simulink model "Flight_Controller_ForStudent"  (R2017b)
settings: Solver=FixedStepDiscrete  StartTime=0.0  StopTime=10.0  FixedStep=Ts  RelTol=1e-3
undefined symbols (not defined in the file or in its folder): Actuators, Gear, Lim, Sim_trimInput, TP_Euler, Ts
libraries: simulink x4
settings Model: Creator=zht  LastModifiedBy=One

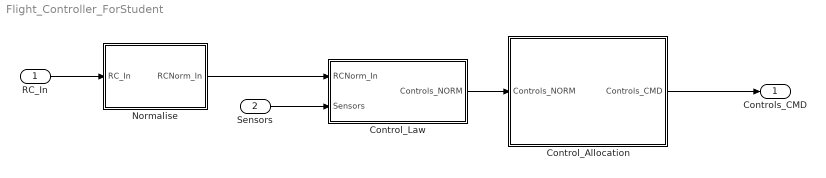
== system Flight_Controller_ForStudent ==
  RC_In : Inport  OutDataTypeStr=Bus: RC_In_BUS
  Sensors : Inport  Port=2  OutDataTypeStr=Bus: Sensors_BUS
  Control_Allocation : Subsystem
  Control_Law : Subsystem
  Normalise : Subsystem
  Controls_CMD : Outport  OutDataTypeStr=Bus: Controls_CMD_BUS
  wires:
  Control_Allocation/1(Controls_CMD) -> Controls_CMD/1
  Control_Law/1(Controls_NORM) -> Control_Allocation/1(Controls_NORM)
  Sensors/1 -> Control_Law/2(Sensors)
  RC_In/1 -> Normalise/1(RC_In)
  Normalise/1(RCNorm_In) -> Control_Law/1(RCNorm_In)

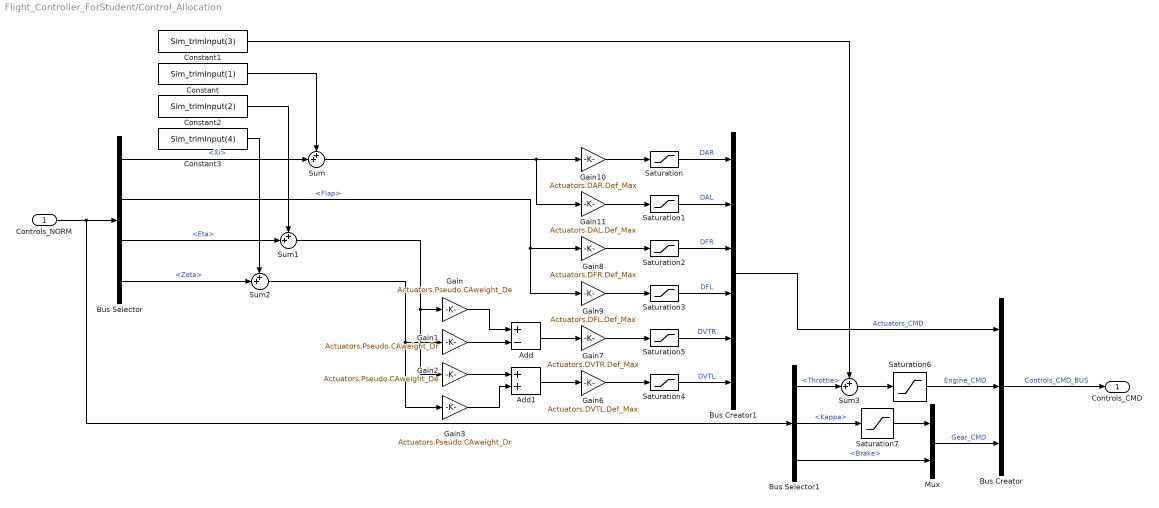
== system Flight_Controller_ForStudent/Control_Allocation ==
  Controls_NORM : Inport
  Add : Sum  Inputs=+-
  Add1 : Sum
  Bus Creator : BusCreator  Inputs=3  OutDataTypeStr=Bus: Controls_CMD_BUS
  Bus Creator1 : BusCreator  Inputs=6  OutDataTypeStr=Bus: Actuators_CMD_BUS
  Bus Selector : BusSelector  OutputSignals=Xi,Flap,Eta,Zeta
  Bus Selector1 : BusSelector  OutputSignals=Throttle,Kappa,Brake
  Constant : Constant  Value=Sim_trimInput(1)
  Constant1 : Constant  Value=Sim_trimInput(3)
  Constant2 : Constant  Value=Sim_trimInput(2)
  Constant3 : Constant  Value=Sim_trimInput(4)
  Gain : Gain  Gain=Actuators.Pseudo.CAweight_De
  Gain1 : Gain  Gain=Actuators.Pseudo.CAweight_Dr
  Gain10 : Gain  Gain=Actuators.DAR.Def_Max
  Gain11 : Gain  Gain=Actuators.DAL.Def_Max
  Gain2 : Gain  Gain=Actuators.Pseudo.CAweight_De
  Gain3 : Gain  Gain=Actuators.Pseudo.CAweight_Dr
  Gain6 : Gain  Gain=Actuators.DVTL.Def_Max
  Gain7 : Gain  Gain=Actuators.DVTR.Def_Max
  Gain8 : Gain  Gain=Actuators.DFR.Def_Max
  Gain9 : Gain  Gain=Actuators.DFL.Def_Max
  Mux : Mux  Inputs=2
  Saturation : Saturate  UpperLimit=Actuators.DAR.Def_Max  LowerLimit=Actuators.DAR.Def_Min
  Saturation1 : Saturate  UpperLimit=Actuators.DAL.Def_Max  LowerLimit=Actuators.DAL.Def_Min
  Saturation2 : Saturate  UpperLimit=Actuators.DFR.Def_Max  LowerLimit=Actuators.DFR.Def_Min
  Saturation3 : Saturate  UpperLimit=Actuators.DAL.Def_Max  LowerLimit=Actuators.DAL.Def_Min
  Saturation4 : Saturate  UpperLimit=Actuators.DVTL.Def_Max  LowerLimit=Actuators.DVTL.Def_Min
  Saturation5 : Saturate  UpperLimit=Actuators.DVTR.Def_Max  LowerLimit=Actuators.DVTR.Def_Min
  Saturation6 : Saturate  UpperLimit=1  LowerLimit=0
  Saturation7 : Saturate  UpperLimit=Gear.NoseStrut.Def_Max  LowerLimit=-Gear.NoseStrut.Def_Max
  Sum{,1..3} (4 alike) : Sum  Inputs=++|
  Controls_CMD : Outport  OutDataTypeStr=Bus: Controls_CMD_BUS
  wires:
  Bus Creator/1 -> Controls_CMD/1  "Controls_CMD_BUS"
  Bus Creator1/1 -> Bus Creator/1  "Actuators_CMD"
  Mux/1 -> Bus Creator/3  "Gear_CMD"
  Controls_NORM/1 -> Bus Selector1/1, Bus Selector/1
  Gain2/1 -> Add1/1
  Gain3/1 -> Add1/2
  Gain1/1 -> Add/2
  Gain/1 -> Add/1
  Saturation/1 -> Bus Creator1/1  "DAR"
  Saturation1/1 -> Bus Creator1/2  "DAL"
  Add/1 -> Gain7/1
  Bus Selector/2 -> Gain8/1, Gain9/1  "<Flap>"
  Saturation2/1 -> Bus Creator1/3  "DFR"
  Saturation3/1 -> Bus Creator1/4  "DFL"
  Add1/1 -> Gain6/1
  Saturation5/1 -> Bus Creator1/5  "DVTR"
  Saturation4/1 -> Bus Creator1/6  "DVTL"
  Saturation6/1 -> Bus Creator/2  "Engine_CMD"
  Bus Selector1/2 -> Saturation7/1  "<Kappa>"
  Bus Selector1/3 -> Mux/2  "<Brake>"
  Saturation7/1 -> Mux/1
  Gain6/1 -> Saturation4/1
  Gain7/1 -> Saturation5/1
  Gain8/1 -> Saturation2/1
  Gain9/1 -> Saturation3/1
  Gain10/1 -> Saturation/1
  Gain11/1 -> Saturation1/1
  Sum/1 -> Gain10/1, Gain11/1
  Sum1/1 -> Gain2/1, Gain/1
  Sum2/1 -> Gain3/1, Gain1/1
  Sum3/1 -> Saturation6/1
  Constant1/1 -> Sum3/1
  Constant2/1 -> Sum1/1
  Constant/1 -> Sum/1
  Constant3/1 -> Sum2/1
  Bus Selector/1 -> Sum/2  "<Xi>"
  Bus Selector/3 -> Sum1/2  "<Eta>"
  Bus Selector/4 -> Sum2/2  "<Zeta>"
  Bus Selector1/1 -> Sum3/2  "<Throttle>"

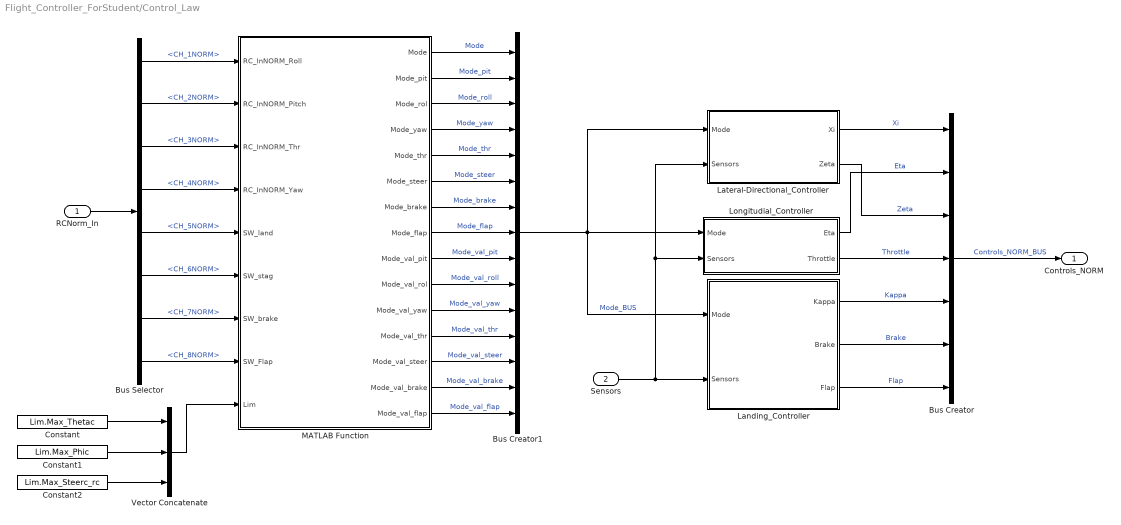
== system Flight_Controller_ForStudent/Control_Law ==
  RCNorm_In : Inport  OutDataTypeStr=Bus: RCNorm_In_BUS
  Sensors : Inport  Port=2  OutDataTypeStr=Bus: Sensors_BUS
  Bus Creator : BusCreator  Inputs=7
  Bus Creator1 : BusCreator  Inputs=15  OutDataTypeStr=Bus: Mode_BUS  NonVirtualBus=on
  Bus Selector : BusSelector  OutputSignals=CH_1NORM,CH_2NORM,CH_3NORM,CH_4NORM,CH_5NORM,CH_6NORM,CH_7NORM,CH_8NORM
  Constant : Constant  Value=Lim.Max_Thetac
  Constant1 : Constant  Value=Lim.Max_Phic
  Constant2 : Constant  Value=Lim.Max_Steerc_rc
  Landing_Controller : Subsystem
  Lateral-Directional_Controller : Subsystem
  Longitudial_Controller : Subsystem
  MATLAB Function : MATLAB Function  TreatAsAtomicUnit=on  SystemSampleTime=Ts
  Vector Concatenate : Concatenate  NumInputs=3
  Controls_NORM : Outport  OutDataTypeStr=Bus: Controls_NORM_BUS
  wires:
  Bus Creator/1 -> Controls_NORM/1  "Controls_NORM_BUS"
  Longitudial_Controller/1(Eta) -> Bus Creator/2  "Eta"
  Lateral-Directional_Controller/2(Zeta) -> Bus Creator/3  "Zeta"
  Lateral-Directional_Controller/1(Xi) -> Bus Creator/1  "Xi"
  Longitudial_Controller/2(Throttle) -> Bus Creator/4  "Throttle"
  Landing_Controller/1(Kappa) -> Bus Creator/5  "Kappa"
  Landing_Controller/2(Brake) -> Bus Creator/6  "Brake"
  Sensors/1 -> Lateral-Directional_Controller/2(Sensors), Longitudial_Controller/2(Sensors), Landing_Controller/2(Sensors)
  RCNorm_In/1 -> Bus Selector/1
  Landing_Controller/3(Flap) -> Bus Creator/7  "Flap"
  Bus Selector/1 -> MATLAB Function/1(RC_InNORM_Roll)  "<CH_1NORM>"
  Bus Selector/2 -> MATLAB Function/2(RC_InNORM_Pitch)  "<CH_2NORM>"
  Bus Selector/3 -> MATLAB Function/3(RC_InNORM_Thr)  "<CH_3NORM>"
  Bus Selector/4 -> MATLAB Function/4(RC_InNORM_Yaw)  "<CH_4NORM>"
  Bus Selector/5 -> MATLAB Function/5(SW_land)  "<CH_5NORM>"
  Bus Selector/6 -> MATLAB Function/6(SW_stag)  "<CH_6NORM>"
  Bus Selector/7 -> MATLAB Function/7(SW_brake)  "<CH_7NORM>"
  Bus Selector/8 -> MATLAB Function/8(SW_Flap)  "<CH_8NORM>"
  MATLAB Function/2(Mode_pit) -> Bus Creator1/2  "Mode_pit"
  MATLAB Function/3(Mode_rol) -> Bus Creator1/3  "Mode_roll"
  MATLAB Function/4(Mode_yaw) -> Bus Creator1/4  "Mode_yaw"
  MATLAB Function/5(Mode_thr) -> Bus Creator1/5  "Mode_thr"
  MATLAB Function/6(Mode_steer) -> Bus Creator1/6  "Mode_steer"
  MATLAB Function/7(Mode_brake) -> Bus Creator1/7  "Mode_brake"
  MATLAB Function/8(Mode_flap) -> Bus Creator1/8  "Mode_flap"
  MATLAB Function/9(Mode_val_pit) -> Bus Creator1/9  "Mode_val_pit"
  MATLAB Function/10(Mode_val_rol) -> Bus Creator1/10  "Mode_val_roll"
  MATLAB Function/11(Mode_val_yaw) -> Bus Creator1/11  "Mode_val_yaw"
  MATLAB Function/12(Mode_val_thr) -> Bus Creator1/12  "Mode_val_thr"
  MATLAB Function/13(Mode_val_steer) -> Bus Creator1/13  "Mode_val_steer"
  MATLAB Function/14(Mode_val_brake) -> Bus Creator1/14  "Mode_val_brake"
  MATLAB Function/15(Mode_val_flap) -> Bus Creator1/15  "Mode_val_flap"
  Bus Creator1/1 -> Lateral-Directional_Controller/1(Mode), Landing_Controller/1(Mode), Longitudial_Controller/1(Mode)  "Mode_BUS"
  MATLAB Function/1(Mode) -> Bus Creator1/1  "Mode"
  Constant/1 -> Vector Concatenate/1
  Constant1/1 -> Vector Concatenate/2
  Constant2/1 -> Vector Concatenate/3
  Vector Concatenate/1 -> MATLAB Function/9(Lim)

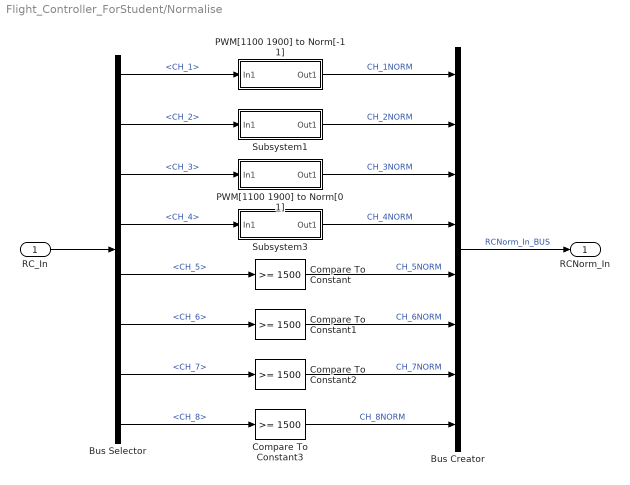
== system Flight_Controller_ForStudent/Normalise ==
  RC_In : Inport  OutDataTypeStr=Bus: RC_In_BUS
  Bus Creator : BusCreator  Inputs=8  OutDataTypeStr=Bus: RCNorm_In_BUS
  Bus Selector : BusSelector  OutputSignals=CH_1,CH_2,CH_3,CH_4,CH_5,CH_6,CH_7,CH_8
  Compare To Constant{,1..3} (4 alike) : simulink/Logic and Bit Operations/Compare To Constant  relop=>=  const=1500  OutDataTypeStr=boolean
  PWM[1100 1900] to Norm[-1 1] : Subsystem
  PWM[1100 1900] to Norm[0 1] : Subsystem
  Subsystem1 : Subsystem
  Subsystem3 : Subsystem
  RCNorm_In : Outport  OutDataTypeStr=Bus: RCNorm_In_BUS
  wires:
  RC_In/1 -> Bus Selector/1
  Bus Selector/1 -> PWM[1100 1900] to Norm[-1 1]/1(In1)  "<CH_1>"
  Bus Selector/2 -> Subsystem1/1(In1)  "<CH_2>"
  Bus Selector/3 -> PWM[1100 1900] to Norm[0 1]/1(In1)  "<CH_3>"
  Bus Selector/4 -> Subsystem3/1(In1)  "<CH_4>"
  Bus Selector/5 -> Compare To Constant/1  "<CH_5>"
  Bus Selector/6 -> Compare To Constant1/1  "<CH_6>"
  Bus Selector/7 -> Compare To Constant2/1  "<CH_7>"
  Bus Selector/8 -> Compare To Constant3/1  "<CH_8>"
  PWM[1100 1900] to Norm[-1 1]/1(Out1) -> Bus Creator/1  "CH_1NORM"
  Subsystem1/1(Out1) -> Bus Creator/2  "CH_2NORM"
  PWM[1100 1900] to Norm[0 1]/1(Out1) -> Bus Creator/3  "CH_3NORM"
  Subsystem3/1(Out1) -> Bus Creator/4  "CH_4NORM"
  Compare To Constant/1 -> Bus Creator/5  "CH_5NORM"
  Compare To Constant1/1 -> Bus Creator/6  "CH_6NORM"
  Compare To Constant2/1 -> Bus Creator/7  "CH_7NORM"
  Compare To Constant3/1 -> Bus Creator/8  "CH_8NORM"
  Bus Creator/1 -> RCNorm_In/1  "RCNorm_In_BUS"

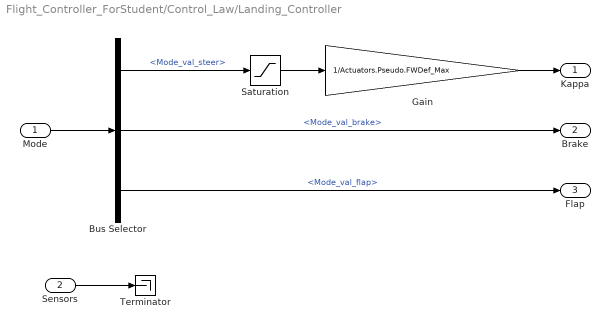
== system Flight_Controller_ForStudent/Control_Law/Landing_Controller ==
  Mode : Inport  OutDataTypeStr=Bus: Mode_BUS
  Sensors : Inport  Port=2  OutDataTypeStr=Bus: Sensors_BUS
  Bus Selector : BusSelector  OutputSignals=Mode_val_steer,Mode_val_brake,Mode_val_flap
  Gain : Gain  Gain=1/Actuators.Pseudo.FWDef_Max
  Saturation : Saturate  UpperLimit=Actuators.Pseudo.FWDef_Max  LowerLimit=-Actuators.Pseudo.FWDef_Max
  Terminator : Terminator
  Kappa : Outport
  Brake : Outport  Port=2
  Flap : Outport  Port=3
  wires:
  Mode/1 -> Bus Selector/1
  Bus Selector/1 -> Saturation/1  "<Mode_val_steer>"
  Bus Selector/2 -> Brake/1  "<Mode_val_brake>"
  Bus Selector/3 -> Flap/1  "<Mode_val_flap>"
  Sensors/1 -> Terminator/1
  Saturation/1 -> Gain/1
  Gain/1 -> Kappa/1

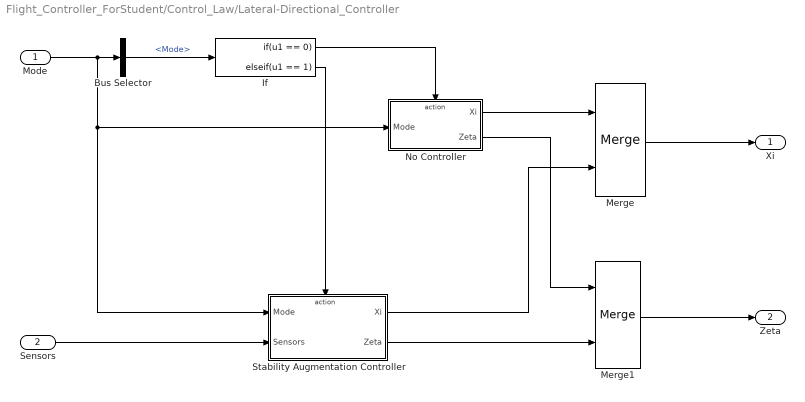
== system Flight_Controller_ForStudent/Control_Law/Lateral-Directional_Controller ==
  Mode : Inport  OutDataTypeStr=Bus: Mode_BUS
  Sensors : Inport  Port=2
  Bus Selector : BusSelector  OutputSignals=Mode
  If : If  IfExpression=u1 == 0  ElseIfExpressions=u1 == 1  ShowElse=off
  Merge : Merge
  Merge1 : Merge
  No Controller : Subsystem  TreatAsAtomicUnit=on
  Stability Augmentation Controller : Subsystem  TreatAsAtomicUnit=on
  Xi : Outport
  Zeta : Outport  Port=2
  wires:
  Sensors/1 -> Stability Augmentation Controller/2(Sensors)
  Mode/1 -> Stability Augmentation Controller/1(Mode), No Controller/1(Mode), Bus Selector/1
  Bus Selector/1 -> If/1  "<Mode>"
  If/1 -> No Controller/Action
  If/2 -> Stability Augmentation Controller/Action
  No Controller/1(Xi) -> Merge/1
  Stability Augmentation Controller/1(Xi) -> Merge/2
  No Controller/2(Zeta) -> Merge1/1
  Stability Augmentation Controller/2(Zeta) -> Merge1/2
  Merge1/1 -> Zeta/1
  Merge/1 -> Xi/1

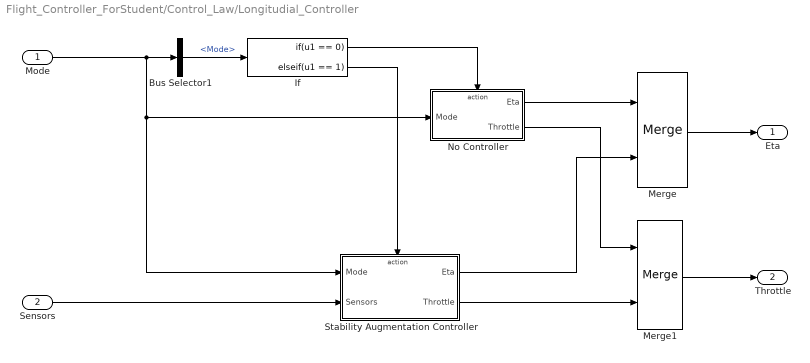
== system Flight_Controller_ForStudent/Control_Law/Longitudial_Controller ==
  Mode : Inport  OutDataTypeStr=Bus: Mode_BUS
  Sensors : Inport  Port=2
  Bus Selector1 : BusSelector  OutputSignals=Mode
  If : If  IfExpression=u1 == 0  ElseIfExpressions=u1 == 1  ShowElse=off
  Merge : Merge
  Merge1 : Merge
  No Controller : Subsystem  TreatAsAtomicUnit=on
  Stability Augmentation Controller : Subsystem  TreatAsAtomicUnit=on
  Eta : Outport
  Throttle : Outport  Port=2
  wires:
  Sensors/1 -> Stability Augmentation Controller/2(Sensors)
  Bus Selector1/1 -> If/1  "<Mode>"
  No Controller/2(Throttle) -> Merge1/1
  If/2 -> Stability Augmentation Controller/Action
  Stability Augmentation Controller/2(Throttle) -> Merge1/2
  If/1 -> No Controller/Action
  Merge1/1 -> Throttle/1
  Merge/1 -> Eta/1
  Mode/1 -> Stability Augmentation Controller/1(Mode), No Controller/1(Mode), Bus Selector1/1
  Stability Augmentation Controller/1(Eta) -> Merge/2
  No Controller/1(Eta) -> Merge/1

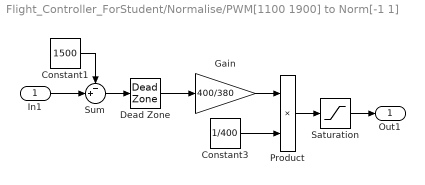
== system Flight_Controller_ForStudent/Normalise/PWM[1100 1900] to Norm[-1 1] ==
  In1 : Inport
  Constant1 : Constant  Value=1500
  Constant3 : Constant  Value=1/400
  Dead Zone : DeadZone  LowerValue=-20  UpperValue=20  SaturateOnIntegerOverflow=on
  Gain : Gain  Gain=400/380
  Product : Product
  Saturation : Saturate  UpperLimit=1  LowerLimit=-1
  Sum : Sum  Inputs=-+|
  Out1 : Outport
  wires:
  Constant3/1 -> Product/2
  Gain/1 -> Product/1
  Product/1 -> Saturation/1
  Sum/1 -> Dead Zone/1
  Constant1/1 -> Sum/1
  Saturation/1 -> Out1/1
  In1/1 -> Sum/2
  Dead Zone/1 -> Gain/1

== system Flight_Controller_ForStudent/Normalise/PWM[1100 1900] to Norm[0 1] ==
  In1 : Inport
  Constant1 : Constant  Value=1100
  Constant3 : Constant  Value=1/780
  Dead Zone : DeadZone  LowerValue=0  UpperValue=20  SaturateOnIntegerOverflow=on
  Product : Product
  Saturation : Saturate  UpperLimit=1  LowerLimit=0
  Sum : Sum  Inputs=-+|
  Out1 : Outport
  wires:
  Constant3/1 -> Product/2
  Dead Zone/1 -> Product/1
  Product/1 -> Saturation/1
  Sum/1 -> Dead Zone/1
  Constant1/1 -> Sum/1
  Saturation/1 -> Out1/1
  In1/1 -> Sum/2

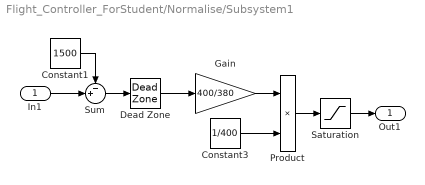
== system Flight_Controller_ForStudent/Normalise/Subsystem1 ==
  In1 : Inport
  Constant1 : Constant  Value=1500
  Constant3 : Constant  Value=1/400
  Dead Zone : DeadZone  LowerValue=-20  UpperValue=20  SaturateOnIntegerOverflow=on
  Gain : Gain  Gain=400/380
  Product : Product
  Saturation : Saturate  UpperLimit=1  LowerLimit=-1
  Sum : Sum  Inputs=-+|
  Out1 : Outport
  wires:
  Dead Zone/1 -> Gain/1
  In1/1 -> Sum/2
  Saturation/1 -> Out1/1
  Constant1/1 -> Sum/1
  Sum/1 -> Dead Zone/1
  Product/1 -> Saturation/1
  Gain/1 -> Product/1
  Constant3/1 -> Product/2

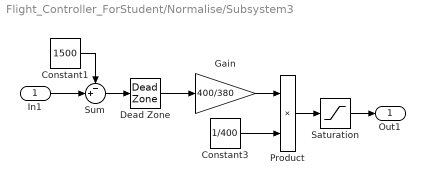
== system Flight_Controller_ForStudent/Normalise/Subsystem3 ==
  In1 : Inport
  Constant1 : Constant  Value=1500
  Constant3 : Constant  Value=1/400
  Dead Zone : DeadZone  LowerValue=-20  UpperValue=20  SaturateOnIntegerOverflow=on
  Gain : Gain  Gain=400/380
  Product : Product
  Saturation : Saturate  UpperLimit=1  LowerLimit=-1
  Sum : Sum  Inputs=-+|
  Out1 : Outport
  wires:
  Dead Zone/1 -> Gain/1
  In1/1 -> Sum/2
  Saturation/1 -> Out1/1
  Constant1/1 -> Sum/1
  Sum/1 -> Dead Zone/1
  Product/1 -> Saturation/1
  Gain/1 -> Product/1
  Constant3/1 -> Product/2

== system Flight_Controller_ForStudent/Control_Law/Lateral-Directional_Controller/No Controller ==
  Mode : Inport  OutDataTypeStr=Bus: Mode_BUS
  Action Port : ActionPort  ActionType=then
  Bus Selector : BusSelector  OutputSignals=Mode_val_roll,Mode_val_yaw
  Gain5 : Gain  Gain=-1
  Gain6 : Gain  Gain=-1
  Xi : Outport
  Zeta : Outport  Port=2
  wires:
  Mode/1 -> Bus Selector/1
  Bus Selector/1 -> Gain6/1  "<Mode_val_roll>"
  Bus Selector/2 -> Gain5/1  "<Mode_val_yaw>"
  Gain6/1 -> Xi/1
  Gain5/1 -> Zeta/1

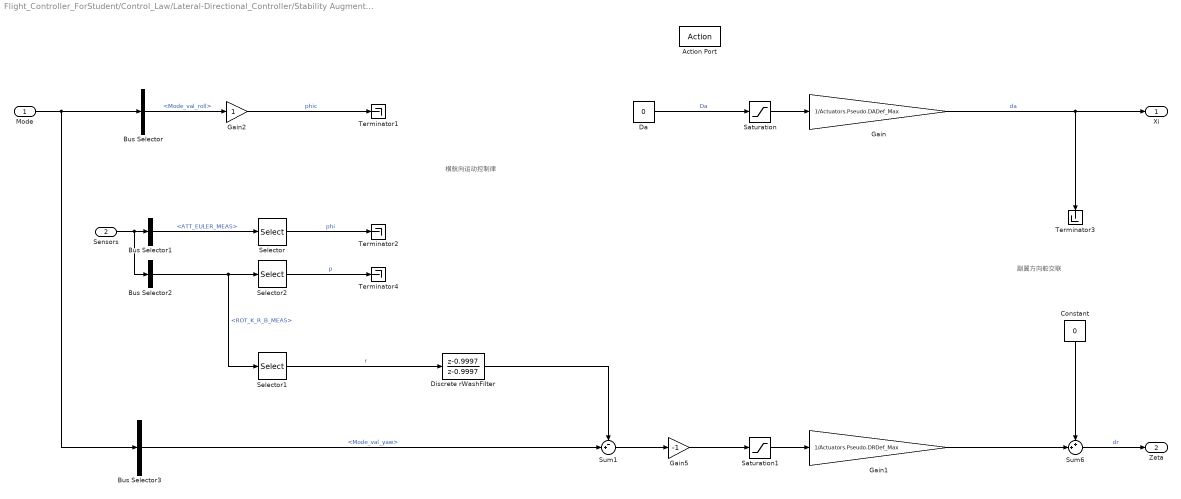
== system Flight_Controller_ForStudent/Control_Law/Lateral-Directional_Controller/Stability Augmentation Controller ==
  note: 横航向运动控制律
  note: 副翼方向舵交联
  Mode : Inport  OutDataTypeStr=Bus: Mode_BUS
  Sensors : Inport  Port=2
  Action Port : ActionPort  ActionType=elseif
  Bus Selector : BusSelector  OutputSignals=Mode_val_roll
  Bus Selector1 : BusSelector  OutputSignals=ATT_EULER_MEAS
  Bus Selector2 : BusSelector  OutputSignals=ROT_K_R_B_MEAS
  Bus Selector3 : BusSelector  OutputSignals=Mode_val_yaw
  Constant : Constant  Value=0
  Da : Constant  Value=0
  Discrete rWashFilter : DiscreteTransferFcn  Numerator=[1 -0.9997]  Denominator=[1 -0.9997]
  Gain : Gain  Gain=1/Actuators.Pseudo.DADef_Max
  Gain1 : Gain  Gain=1/Actuators.Pseudo.DRDef_Max
  Gain2 : Gain
  Gain5 : Gain  Gain=-1
  Saturation : Saturate  UpperLimit=Actuators.Pseudo.DADef_Max  LowerLimit=-Actuators.Pseudo.DADef_Max
  Saturation1 : Saturate  UpperLimit=Actuators.Pseudo.DRDef_Max  LowerLimit=-Actuators.Pseudo.DRDef_Max
  Selector : Selector  InputPortWidth=3  IndexOptions=Index vector (dialog)  Indices=[1]  OutputSizes=1
  Selector1 : Selector  InputPortWidth=3  IndexOptions=Index vector (dialog)  Indices=[3]  OutputSizes=1
  Selector2 : Selector  InputPortWidth=3  IndexOptions=Index vector (dialog)  Indices=[1]  OutputSizes=1
  Sum1 : Sum  Inputs=-+|
  Sum6 : Sum  Inputs=++|
  Terminator{1..4} (4 alike) : Terminator
  Xi : Outport
  Zeta : Outport  Port=2
  wires:
  Bus Selector/1 -> Gain2/1  "<Mode_val_roll>"
  Mode/1 -> Bus Selector3/1, Bus Selector/1
  Saturation/1 -> Gain/1
  Saturation1/1 -> Gain1/1
  Sensors/1 -> Bus Selector2/1, Bus Selector1/1
  Bus Selector1/1 -> Selector/1  "<ATT_EULER_MEAS>"
  Selector1/1 -> Discrete rWashFilter/1  "r"
  Constant/1 -> Sum6/1
  Bus Selector2/1 -> Selector2/1, Selector1/1  "<ROT_K_R_B_MEAS>"
  Sum1/1 -> Gain5/1
  Gain5/1 -> Saturation1/1
  Gain1/1 -> Sum6/2
  Gain/1 -> Xi/1, Terminator3/1  "da"
  Sum6/1 -> Zeta/1  "dr"
  Da/1 -> Saturation/1  "Da"
  Selector2/1 -> Terminator4/1  "p"
  Discrete rWashFilter/1 -> Sum1/1
  Bus Selector3/1 -> Sum1/2  "<Mode_val_yaw>"
  Selector/1 -> Terminator2/1  "phi"
  Gain2/1 -> Terminator1/1  "phic"

== system Flight_Controller_ForStudent/Control_Law/Longitudial_Controller/No Controller ==
  Mode : Inport  OutDataTypeStr=Bus: Mode_BUS
  Action Port : ActionPort  ActionType=then
  Bus Selector : BusSelector  OutputSignals=Mode_val_pit,Mode_val_thr
  Gain3 : Gain  Gain=-1
  Eta : Outport
  Throttle : Outport  Port=2
  wires:
  Mode/1 -> Bus Selector/1
  Bus Selector/1 -> Gain3/1  "<Mode_val_pit>"
  Bus Selector/2 -> Throttle/1  "<Mode_val_thr>"
  Gain3/1 -> Eta/1

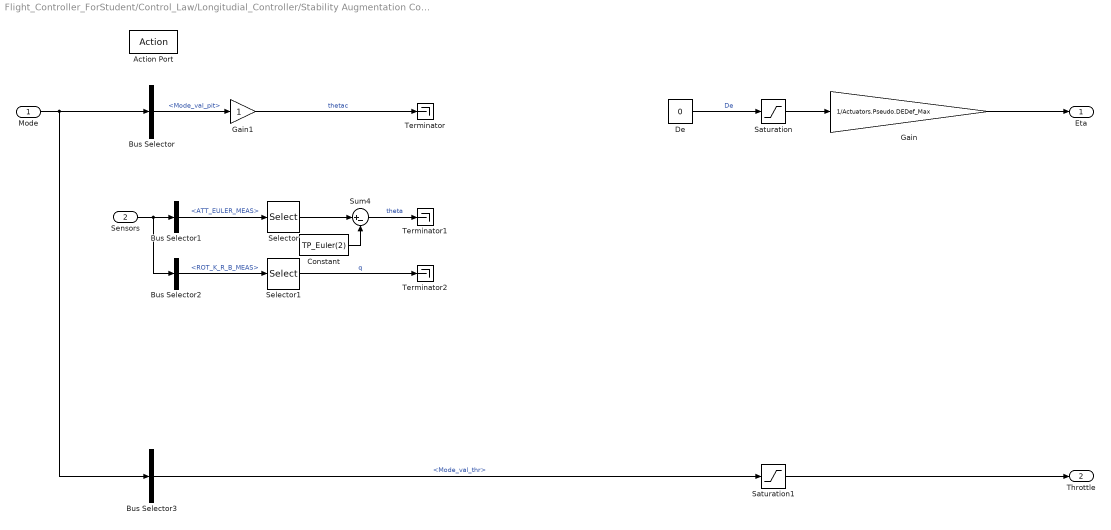
== system Flight_Controller_ForStudent/Control_Law/Longitudial_Controller/Stability Augmentation Controller ==
  Mode : Inport  OutDataTypeStr=Bus: Mode_BUS
  Sensors : Inport  Port=2
  Action Port : ActionPort  ActionType=elseif
  Bus Selector : BusSelector  OutputSignals=Mode_val_pit
  Bus Selector1 : BusSelector  OutputSignals=ATT_EULER_MEAS
  Bus Selector2 : BusSelector  OutputSignals=ROT_K_R_B_MEAS
  Bus Selector3 : BusSelector  OutputSignals=Mode_val_thr
  Constant : Constant  Value=TP_Euler(2)
  De : Constant  Value=0
  Gain : Gain  Gain=1/Actuators.Pseudo.DEDef_Max
  Gain1 : Gain
  Saturation : Saturate  UpperLimit=Actuators.Pseudo.DEDef_Max  LowerLimit=-Actuators.Pseudo.DEDef_Max
  Saturation1 : Saturate  UpperLimit=1  LowerLimit=0
  Selector : Selector  InputPortWidth=3  IndexOptions=Index vector (dialog)  Indices=[2]  OutputSizes=1
  Selector1 : Selector  InputPortWidth=3  IndexOptions=Index vector (dialog)  Indices=[2]  OutputSizes=1
  Sum4 : Sum  Inputs=|+-
  Terminator : Terminator
  Terminator1 : Terminator
  Terminator2 : Terminator
  Eta : Outport
  Throttle : Outport  Port=2
  wires:
  Mode/1 -> Bus Selector/1, Bus Selector3/1
  Saturation/1 -> Gain/1
  Saturation1/1 -> Throttle/1
  Sensors/1 -> Bus Selector2/1, Bus Selector1/1
  Bus Selector1/1 -> Selector/1  "<ATT_EULER_MEAS>"
  Selector/1 -> Sum4/1
  Bus Selector2/1 -> Selector1/1  "<ROT_K_R_B_MEAS>"
  Gain/1 -> Eta/1
  Constant/1 -> Sum4/2
  Bus Selector3/1 -> Saturation1/1  "<Mode_val_thr>"
  De/1 -> Saturation/1  "De"
  Bus Selector/1 -> Gain1/1  "<Mode_val_pit>"
  Sum4/1 -> Terminator1/1  "theta"
  Selector1/1 -> Terminator2/1  "q"
  Gain1/1 -> Terminator/1  "thetac"

== matlab function Flight_Controller_ForStudent/Control_Law/MATLAB Function ==
  data: RC_InNORM_Roll input; Mode output; RC_InNORM_Pitch input; RC_InNORM_Thr input; RC_InNORM_Yaw input; SW_land input; SW_stag input; SW_brake input; SW_Flap input; Lim input; Mode_pit output; Mode_rol output; Mode_yaw output; Mode_thr output; Mode_steer output; Mode_brake output; Mode_flap output; Mode_val_pit output; Mode_val_rol output; Mode_val_yaw output; Mode_val_thr output; Mode_val_steer output; Mode_val_brake output; Mode_val_flap output
function [Mode,Mode_pit,Mode_rol,Mode_yaw,Mode_thr,Mode_steer,Mode_brake,Mode_flap,Mode_val_pit,Mode_val_rol,Mode_val_yaw,Mode_val_thr,Mode_val_steer, Mode_val_brake,Mode_val_flap]      =      ModeManager(RC_InNORM_Roll,RC_InNORM_Pitch,RC_InNORM_Thr,RC_InNORM_Yaw,SW_land,SW_stag,SW_brake,SW_Flap,Lim)

Max_Thetac      = Lim(1);
Max_Phic        = Lim(2);
Max_Steerc_rc   = Lim(3);

%% initialize
Mode            = int8(0);
Mode_pit        = int8(0);
Mode_rol        = int8(0);
Mode_yaw        = int8(0);
Mode_thr        = int8(0);
Mode_steer      = int8(0);                                                  %为地面模型留出接口
Mode_brake      = int8(0);
Mode_flap       = int8(0);

Mode_val_pit    = 0;
Mode_val_rol    = 0;
Mode_val_yaw    = 0;
Mode_val_thr    = 0;
Mode_val_steer  = 0;
Mode_val_flap   = 0;
Mode_val_brake  = 0;

%% judge mode
%默认情况：增稳模式 关
Mode = int8(0);
Mode_val_pit   = RC_InNORM_Pitch;
Mode_val_rol   = RC_InNORM_Roll;
Mode_val_yaw   = RC_InNORM_Yaw;
Mode_val_thr   = RC_InNORM_Thr;
Mode_val_steer = RC_InNORM_Yaw;
if SW_Flap == 1
    Mode_flap = int8(1);
    Mode_val_flap = 1;
end


if (SW_stag == 1) %增稳模式 开
    Mode = int8(1);
    
    Mode_val_pit = RC_InNORM_Pitch*Max_Thetac;
    Mode_val_rol = RC_InNORM_Roll*Max_Phic;
    Mode_val_yaw = RC_InNORM_Yaw*Max_Steerc_rc;                               % [rad/s]
    %Mode_val_thr = Mode_stag_Vc_Min+RC_InNORM_Thr*(Mode_stag_Vc_Max-Mode_stag_Vc_Min);
    Mode_val_thr = RC_InNORM_Thr;
    Mode_val_steer = RC_InNORM_Yaw*Max_Steerc_rc;                             % [rad/s]
    if SW_Flap == 1
        Mode_flap = int8(1);
        Mode_val_flap = 1;
    end
end
end
